simulink model "Ball_following_angular_1"  (R2021a)
settings: Solver=VariableStepAuto  StartTime=0.0  StopTime=inf  RelTol=1e-3
libraries: mobileRoboticsLib x6
settings Model: Creator=its_ghani  LastModifiedBy=its_ghani

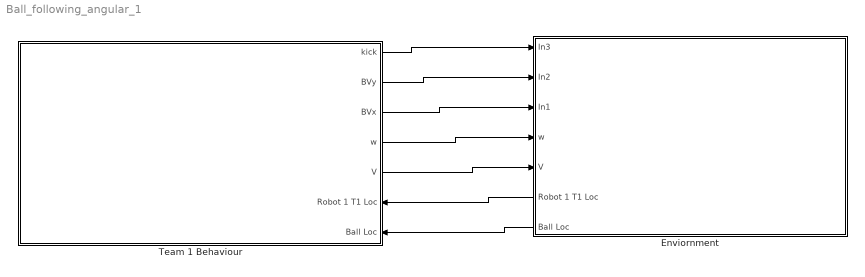
== system Ball_following_angular_1 ==
  Enviornment : Subsystem
      settings: PortSchema="{\"entries\":[{\"content\":{\"sides\":[{\"content\":{\"connectorIds\":[\"In1\",\"In2\",\"In3\",\"In4\",\"In5\",\"Out1\",\"Out2\"]},\"type\":\"ConnectorPlacement.EquallySpacedRectSide\",\"uuid\":\"bfc4f995-18bb-40a5-813e-439d500b4bf9\"},{\"content\":{\"connectorIds\":[],\"side\":\"RIGHT\"},\"type\":\"ConnectorPlacement.EquallySpacedRectSide\",\"uuid\":\"3fb6b8a6-16df-4a59-8ba5-6321e26d1fdd\"},{\"content\":{\"connectorIds\":[],\"side\":\"TOP\"},\"type\":\"ConnectorPlacement.EquallySpacedRectSide\",\"uuid\":\"a9e4cd1b-3afe-4395-99fa-15aef12a4070\"}]},\"type\":\"ConnectorPlacement.EquallySpacedConnector\",\"uuid\":\"a6ca697e-fe67-43ac-b669-91f3e6c836c9\"}],\"packageUris\":[\"http://schema.mathworks.com/mf0/Connector/R2020b\"],\"version\":\"1.0\"}"
  Team 1 Behaviour : Subsystem
      settings: PortSchema="{\"entries\":[{\"content\":{\"sides\":[{\"content\":{\"connectorIds\":[]},\"type\":\"ConnectorPlacement.EquallySpacedRectSide\",\"uuid\":\"be901545-21b9-45e5-bac5-a8cb9027aef5\"},{\"content\":{\"connectorIds\":[\"Out1\",\"Out2\",\"Out3\",\"Out4\",\"Out5\",\"In1\",\"In2\"],\"side\":\"RIGHT\"},\"type\":\"ConnectorPlacement.EquallySpacedRectSide\",\"uuid\":\"b7c1eb84-2f14-4c7f-a74c-d56efbe0743e\"},{\"content\":{\"connectorIds\":[],\"side\":\"TOP\"},\"type\":\"ConnectorPlacement.EquallySpacedRectSide\",\"uuid\":\"aca41723-ed3f-4bd2-8fc1-457d075e3460\"}]},\"type\":\"ConnectorPlacement.EquallySpacedConnector\",\"uuid\":\"e10e22f1-c8f0-4dfc-85d2-4ba01528372d\"}],\"packageUris\":[\"http://schema.mathworks.com/mf0/Connector/R2020b\"],\"version\":\"1.0\"}"
  wires:
  Team 1 Behaviour/5("V\t") -> Enviornment/5(V)
  Enviornment/1(Robot 1 T1 Loc) -> Team 1 Behaviour/1(Robot 1 T1 Loc)
  Enviornment/2(Ball Loc) -> Team 1 Behaviour/2(Ball Loc)
  Team 1 Behaviour/4(w) -> Enviornment/4(w)
  Team 1 Behaviour/3(BVx) -> Enviornment/3(In1)
  Team 1 Behaviour/2(BVy) -> Enviornment/2(In2)
  Team 1 Behaviour/1(kick) -> Enviornment/1(In3)

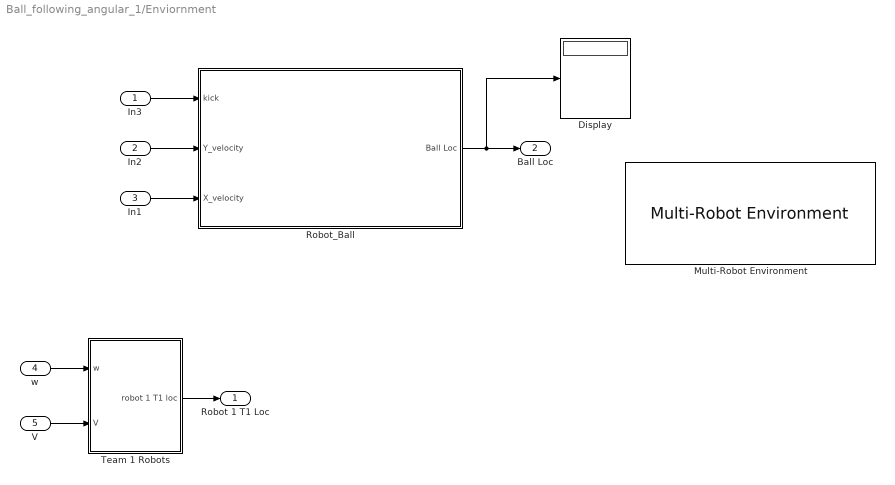
== system Ball_following_angular_1/Enviornment ==
  In3 : Inport
  In2 : Inport  Port=2
  In1 : Inport  Port=3
  w : Inport  Port=4
  V : Inport  Port=5
  "\tTeam 1 Robots" : Subsystem
  Display : Display
  Multi-Robot Environment : mobileRoboticsLib/Environments/Multi-Robot Environment  numRobots=2  showWaypoints=off  showObjects=off  objectColors=[1 0 0;0 1 0;0 0 1]  objectMarkers='s'  showRobotIds=on  plotSensorLines=off
      settings: SourceProductName=Mobile Robotics Simulation Toolbox
  Robot_Ball : Subsystem
  Robot 1 T1 Loc : Outport
  Ball Loc : Outport  Port=2
  wires:
  "\tTeam 1 Robots"/1(robot 1 T1 loc) -> Robot 1 T1 Loc/1
  V/1 -> "\tTeam 1 Robots"/2(V)
  w/1 -> "\tTeam 1 Robots"/1(w)
  In2/1 -> Robot_Ball/2(Y_velocity)
  In1/1 -> Robot_Ball/3(X_velocity)
  Robot_Ball/1(Ball Loc) -> Display/1, Ball Loc/1
  In3/1 -> Robot_Ball/1(kick)

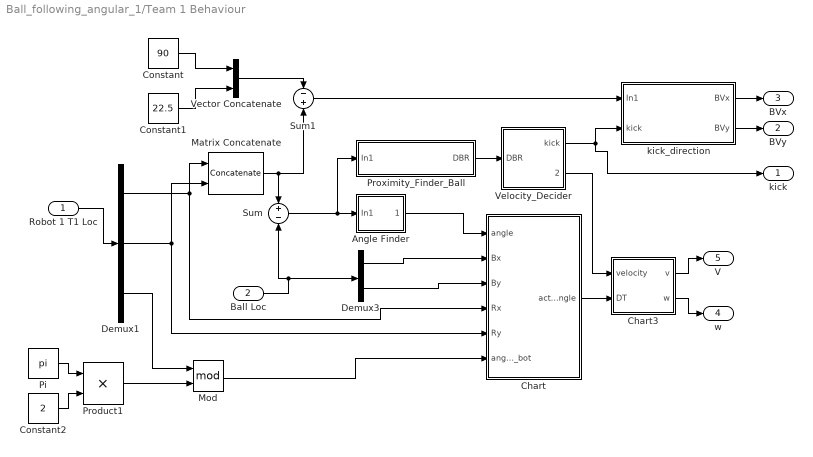
== system Ball_following_angular_1/Team 1 Behaviour ==
  Robot 1 T1 Loc : Inport
  Ball Loc : Inport  Port=2
  Angle Finder : Subsystem
  Chart : Stateflow chart  TreatAsAtomicUnit=on
      settings: PortSchema="{\"entries\":[{\"content\":{\"sides\":[{\"content\":{\"connectorIds\":[\"In5\",\"In1\",\"In2\",\"In3\",\"In4\",\"In6\"]},\"type\":\"ConnectorPlacement.EquallySpacedRectSide\",\"uuid\":\"cd25ea97-6441-4246-83f2-eec847899c89\"},{\"content\":{\"connectorIds\":[\"Out1\"],\"side\":\"RIGHT\"},\"type\":\"ConnectorPlacement.EquallySpacedRectSide\",\"uuid\":\"ef7d77a7-1549-4474-8b84-35bb8af5d0e7\"},{\"content\":{\"connectorIds\":[],\"side\":\"TOP\"},\"type\":\"ConnectorPlacement.EquallySpacedRectSide\",\"uuid\":\"0f0ce596-3061-42ac-890a-62bc4f21ac3e\"},{\"content\":{\"connectorIds\":[],\"side\":\"BOTTOM\"},\"type\":\"ConnectorPlacement.EquallySpacedRectSide\",\"uuid\":\"682b3de5-e999-4954-b7ff-f16ecbf9ea8f\"}]},\"type\":\"ConnectorPlacement.EquallySpacedConnector\",\"uuid\":\"15dca8e2-6a60-4a0d-80a5-3c295a61c828\"}],\"packageUris\":[\"http://schema.mathworks.com/mf0/Connector/R2020b\"],\"version\":\"1.0\"}"
  Chart3 : Stateflow chart  TreatAsAtomicUnit=on
  Constant : Constant  Value=90
  Constant1 : Constant  Value=22.5
  Constant2 : Constant  Value=2
  Demux1 : Demux  Outputs=3
  Demux3 : Demux  Outputs=2
  Matrix Concatenate : Concatenate  Mode=Multidimensional array  ConcatenateDimension=2
  Mod : Math  Operator=mod  SaturateOnIntegerOverflow=on
  Pi : Constant  Value=pi  OutDataTypeStr=Inherit: Inherit via back propagation
  Product1 : Product
  Proximity_Finder_Ball : Subsystem
  Sum : Sum  Inputs=+-
  Sum1 : Sum  Inputs=-+
  Vector Concatenate : Concatenate
  Velocity_Decider : Stateflow chart  TreatAsAtomicUnit=on
  kick_direction : Subsystem
  kick : Outport
  BVy : Outport  Port=2
  BVx : Outport  Port=3
  w : Outport  Port=4
  "V\t" : Outport  Port=5
  wires:
  Ball Loc/1 -> Sum/2, Demux3/1
  Sum/1 -> Proximity_Finder_Ball/1(In1), Angle Finder/1(In1)
  Robot 1 T1 Loc/1 -> Demux1/1
  Demux1/1 -> Matrix Concatenate/1, Chart/3(Rx)
  Demux1/2 -> Matrix Concatenate/2, Chart/4(Ry)
  Matrix Concatenate/1 -> Sum1/2, Sum/1
  Chart3/2(w) -> w/1
  Chart3/1(v) -> "V\t"/1
  Demux3/2 -> Chart/2(By)
  Demux3/1 -> Chart/1(Bx)
  Demux1/3 -> Mod/1
  Pi/1 -> Product1/1
  Constant2/1 -> Product1/2
  Product1/1 -> Mod/2
  Chart/1(actual_angle) -> Chart3/2(DT)
  Mod/1 -> Chart/6(angle_bot)
  Angle Finder/1(angle) -> Chart/5(angle)
  Proximity_Finder_Ball/1(DBR) -> Velocity_Decider/1(DBR)
  Velocity_Decider/2(velocity) -> Chart3/1(velocity)
  Constant/1 -> Vector Concatenate/1
  Constant1/1 -> Vector Concatenate/2
  Vector Concatenate/1 -> Sum1/1
  Sum1/1 -> kick_direction/1(In1)
  Velocity_Decider/1(kick) -> kick/1, kick_direction/2(kick)
  kick_direction/1(BVx) -> BVx/1
  kick_direction/2(BVy) -> BVy/1

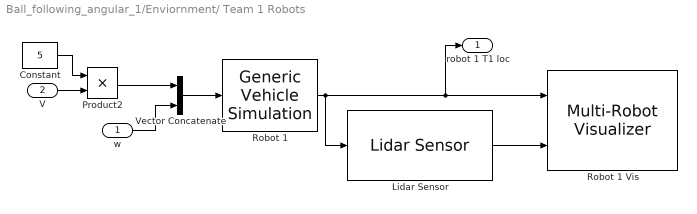
== system Ball_following_angular_1/Enviornment/	Team 1 Robots ==
  w : Inport
  V : Inport  Port=2
  Constant : Constant  Value=5
  Lidar Sensor : mobileRoboticsLib/Environments/Lidar Sensor  sensorOffset=[ 0, 0 ]  scanAngles=[ -pi/4, 0, pi/4 ]  maxRange=5  isMultiRobot=on  robotIdx=1
      settings: SourceProductName=Mobile Robotics Simulation Toolbox
  Product2 : Product
  Robot 1 : mobileRoboticsLib/Utilities/Generic Vehicle Simulation  initX=0  initY=45  initAngle=0  Ts=0.05
      settings: SourceProductName=Mobile Robotics Simulation Toolbox
  Robot 1 Vis : mobileRoboticsLib/Environments/Multi-Robot Visualizer  idx=1  radius=1  robotColor=[0 0 1]  showTraj=on  hasLidar=on  sensorOffset=[0,0]  scanAngles=[-pi/4, 0, pi/4]  hasObjDetector=off  objDetectorOffset=[0,0]  objDetectorAngle=0  objDetectorFOV=pi/3  objDetectorMaxRange=5
      settings: SourceProductName=Mobile Robotics Simulation Toolbox
  Vector Concatenate : Concatenate  NumInputs=3
  robot 1 T1 loc : Outport
  wires:
  Vector Concatenate/1 -> Robot 1/1
  Robot 1/1 -> robot 1 T1 loc/1, Robot 1 Vis/1, Lidar Sensor/1
  Lidar Sensor/1 -> Robot 1 Vis/2
  w/1 -> Vector Concatenate/3
  Product2/1 -> Vector Concatenate/1
  V/1 -> Product2/2
  Constant/1 -> Product2/1

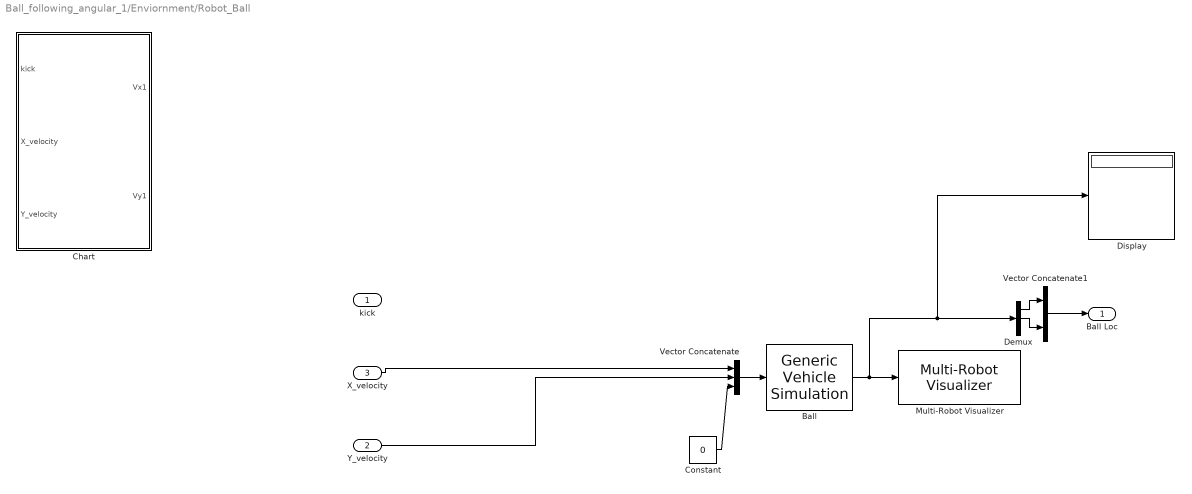
== system Ball_following_angular_1/Enviornment/Robot_Ball ==
  kick : Inport
  Y_velocity : Inport  Port=2
  X_velocity : Inport  Port=3
  Ball : mobileRoboticsLib/Utilities/Generic Vehicle Simulation  initX=45  initY=22.5  initAngle=0  Ts=0.05
      settings: SourceProductName=Mobile Robotics Simulation Toolbox
  Chart : Stateflow chart  TreatAsAtomicUnit=on
  Constant : Constant  Value=0
  Demux : Demux  Outputs=3
  Display : Display
  Multi-Robot Visualizer : mobileRoboticsLib/Environments/Multi-Robot Visualizer  idx=2  radius=0  robotColor=[0 1 1]  showTraj=off  hasLidar=off  sensorOffset=[0,0]  scanAngles=[-pi/4, 0, pi/4]  hasObjDetector=off  objDetectorOffset=[0,0]  objDetectorAngle=0  objDetectorFOV=pi/3  objDetectorMaxRange=5
      settings: SourceProductName=Mobile Robotics Simulation Toolbox
  Vector Concatenate : Concatenate  NumInputs=3
  Vector Concatenate1 : Concatenate
  Ball Loc : Outport
  wires:
  Demux/2 -> Vector Concatenate1/2
  Demux/1 -> Vector Concatenate1/1
  Vector Concatenate1/1 -> Ball Loc/1
  Constant/1 -> Vector Concatenate/3
  Vector Concatenate/1 -> Ball/1
  Ball/1 -> Display/1, Demux/1, Multi-Robot Visualizer/1
  X_velocity/1 -> Vector Concatenate/1
  Y_velocity/1 -> Vector Concatenate/2

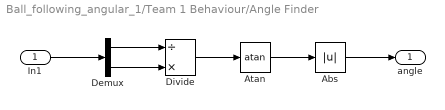
== system Ball_following_angular_1/Team 1 Behaviour/Angle Finder ==
  In1 : Inport
  Abs : Abs
  Atan : Trigonometry  Operator=atan
  Demux : Demux  Outputs=2
  Divide : Product  Inputs=/*
  angle : Outport
  wires:
  Divide/1 -> Atan/1
  Demux/2 -> Divide/2
  Demux/1 -> Divide/1
  Atan/1 -> Abs/1
  Abs/1 -> angle/1
  In1/1 -> Demux/1

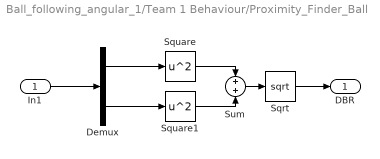
== system Ball_following_angular_1/Team 1 Behaviour/Proximity_Finder_Ball ==
  In1 : Inport
  Demux : Demux  Outputs=2
  Sqrt : Sqrt  SaturateOnIntegerOverflow=on
  Square : Math  Operator=square  SaturateOnIntegerOverflow=on
  Square1 : Math  Operator=square  SaturateOnIntegerOverflow=on
  Sum : Sum
  DBR : Outport
  wires:
  In1/1 -> Demux/1
  Demux/1 -> Square/1
  Demux/2 -> Square1/1
  Square1/1 -> Sum/2
  Square/1 -> Sum/1
  Sum/1 -> Sqrt/1
  Sqrt/1 -> DBR/1

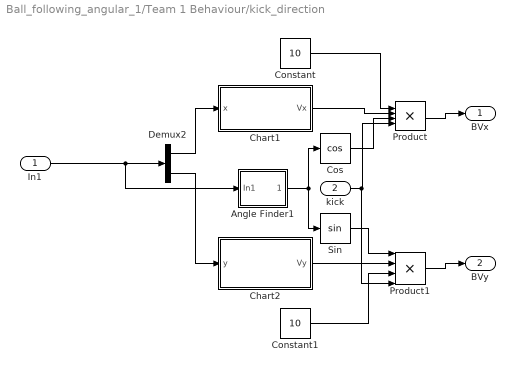
== system Ball_following_angular_1/Team 1 Behaviour/kick_direction ==
  In1 : Inport
  kick : Inport  Port=2
  Angle Finder1 : Subsystem
  Chart1 : Stateflow chart  TreatAsAtomicUnit=on
  Chart2 : Stateflow chart  TreatAsAtomicUnit=on
  Constant : Constant  Value=10
  Constant1 : Constant  Value=10
  Cos : Trigonometry  Operator=cos
  Demux2 : Demux  Outputs=2
  Product : Product  Inputs=4
  Product1 : Product  Inputs=4
  Sin : Trigonometry
  BVx : Outport
  BVy : Outport  Port=2
  wires:
  Demux2/2 -> Chart2/1(y)
  Demux2/1 -> Chart1/1(x)
  In1/1 -> Angle Finder1/1(In1), Demux2/1
  Chart1/1(Vx) -> Product/2
  Cos/1 -> Product/3
  Angle Finder1/1(angle) -> Cos/1, Sin/1
  Constant/1 -> Product/1
  Product/1 -> BVx/1
  Product1/1 -> BVy/1
  Constant1/1 -> Product1/3
  Chart2/1(Vy) -> Product1/2
  Sin/1 -> Product1/1
  kick/1 -> Product1/4, Product/4

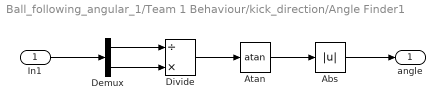
== system Ball_following_angular_1/Team 1 Behaviour/kick_direction/Angle Finder1 ==
  In1 : Inport
  Abs : Abs
  Atan : Trigonometry  Operator=atan
  Demux : Demux  Outputs=2
  Divide : Product  Inputs=/*
  angle : Outport
  wires:
  Divide/1 -> Atan/1
  Demux/2 -> Divide/2
  Demux/1 -> Divide/1
  Atan/1 -> Abs/1
  Abs/1 -> angle/1
  In1/1 -> Demux/1

== stateflow chart Ball_following_angular_1/Team 1 Behaviour/kick_direction/Chart1 ==
  state x_pos
    du:
    Vx = 1
  state x_neg
    du:
    Vx = -1
  (default) -> x_pos
  x_pos -> x_neg : [x > 0]
  x_neg -> x_pos : [x<1]
  data: Vx output; x input

== stateflow chart Ball_following_angular_1/Team 1 Behaviour/kick_direction/Chart2 ==
  state y_pos
    du:
    Vy = 1
  state y_neg
    du:
    Vy = -1
  (default) -> y_pos
  y_pos -> y_neg : [y > 0]
  y_neg -> y_pos : [y<1]
  data: y input; Vy output

== stateflow chart Ball_following_angular_1/Team 1 Behaviour/Velocity_Decider ==
  state Robot_Far
    du:
    velocity = 1;
    kick = 0;
  state Robot_Close
    du:
    velocity = 0;
    kick = 1;
  (default) -> Robot_Far
  Robot_Far -> Robot_Close : [DBR <= 0.25]
  Robot_Close -> Robot_Far : [DBR > 0.25]
  data: kick output; DBR input; velocity output

== stateflow chart Ball_following_angular_1/Team 1 Behaviour/Chart ==
  state second_coordinate
    du:
    actual_angle = -pi +angle + angle_bot;
  state first_coordinate
    du:
    actual_angle = angle_bot - angle;
  state ffourth_coordinate
    du:
    actual_angle = -(2*pi) + angle + angle_bot
  state Third_coordinate
    du:
    actual_angle =-(pi) - angle + angle_bot;
  (default) -> first_coordinate
  first_coordinate -> second_coordinate [order 1] : [ Rx>Bx && Ry<By ]
  second_coordinate -> first_coordinate [order 1] : [ Rx<Bx && Ry<By]
  ffourth_coordinate -> second_coordinate [order 1] : [ Rx>Bx && Ry<By ]
  first_coordinate -> Third_coordinate [order 3] : [ Rx>Bx && Ry>By]
  second_coordinate -> Third_coordinate [order 3] : [ Rx>Bx && Ry>By ]
  Third_coordinate -> second_coordinate [order 1] : [ Rx>Bx && Ry<By ]
  second_coordinate -> ffourth_coordinate [order 2] : [ Rx<Bx && Ry>By ]
  Third_coordinate -> first_coordinate [order 2] : [ Rx<Bx && Ry<By ]
  ffourth_coordinate -> first_coordinate [order 2] : [ Rx<Bx && Ry<By ]
  first_coordinate -> ffourth_coordinate [order 2] : [ Rx<Bx && Ry>By ]
  Third_coordinate -> ffourth_coordinate [order 3] : [ Rx<Bx && Ry>By ]
  ffourth_coordinate -> Third_coordinate [order 3] : [ Rx>Bx && Ry>By]
  data: Bx input; By input; Rx input; Ry input; angle input; actual_angle output; angle_bot input

== stateflow chart Ball_following_angular_1/Team 1 Behaviour/Chart3 ==
  state stop
    du:
    w = 0;
    v=1 * velocity;
  state RCW
    du:
    w = -1*1;
    v=0;
  state RCCW
    du:
    w =1*1;
    v=0;
  (default) -> stop
  stop -> RCCW [order 2] : [after(1,sec) && DT > 0]
  stop -> RCW [order 1] : [after(1,sec) && DT < 0]
  RCW -> stop [order 1] : [DT<= 0.1 && DT>= -0.1]
  RCCW -> stop [order 1] : [DT<= 0.1 && DT>= -0.1]
  RCCW -> RCW [order 2] : [DT>0]
  RCW -> RCCW [order 2] : [DT<0]
  data: velocity input; v output; DT input; w output

== stateflow chart Ball_following_angular_1/Enviornment/Robot_Ball/Chart ==
  state Damping
    du:
    if (Vx > 0)
    while(Vx ~= 0)
    Vx = Vx - 0.05;
    Vx1 = Vx
    end
    end
    if (Vx<0)
    while(Vx ~= 0)
    Vx = Vx + 0.05;
    Vx1 = Vx
    end
    end
    if (Vy > 0)
    while(Vy ~= 0)
    Vy = Vy - 0.05;
    Vy1 = Vy
    end
    end
    if (Vy<0)
    while(Vx ~= 0)
    Vy = Vy + 0.05;
    Vy1 = Vy
    end
    end
  state Start
    en:
    Vx = 0
    Vy = 0
  state Kicked
    du:
    Vx = X_velocity
    Vy = Y_velocity
  (default) -> Start
  Start -> Kicked : [kick == 1]
  Kicked -> Damping : [kick == 1]
  Damping -> Kicked : [kick == 1]
  data: kick input; X_velocity input; Y_velocity input; Vx local; Vy local; Vx1 output; Vy1 output
